simulink model "fig7_63_controleffort"  (Simulink 7.0)
settings: Solver=ode45  SolverMode=SingleTasking  StartTime=0.0  StopTime=25  RelTol=1e-3  AbsTol=1e-6
CloseFcn:
  | ;slview('closediagram',bdroot);;slview('closediagram',bdroot);
settings Model: Creator=abbas  LastModifiedBy=abbas  ExtModeTrigMode=oneshot  ExtModeArmWhenConnect=off  ExtModeAutoUpdateStatusClock=off
settings DataIOCC: LimitDataPoints=off
settings OptimizationCC: BlockReduction=off  BooleanDataType=off  InlineInvariantSignals=on
settings DebuggingCC: SaveWithParameterizedLinksMsg=none  SignalResolutionControl=TryResolveAllWithWarning  SolverPrmCheckMsg=none  MultiTaskDSMMsg=warning  MultiTaskCondExecSysMsg=none  StrictBusMsg=None
settings HardwareCC: TargetUnknown=on
settings RTWCC: IncludeERTFirstTime=on
settings GRTTargetCC: TargetFcnLib=ansi_tfl_tmw.mat  ModelReferenceCompliant=off  CompOptLevelCompliant=off  MatFileLogging=off

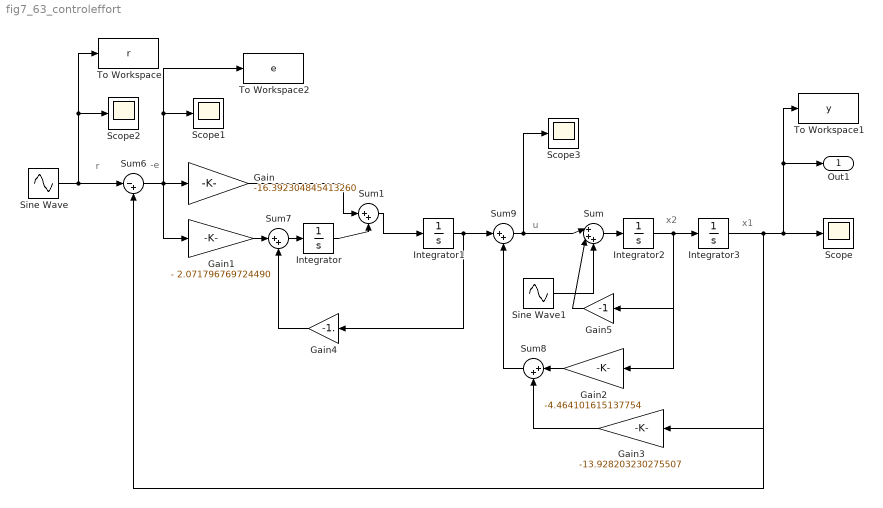
== system fig7_63_controleffort ==
  note: -e
  note: u
  note: x2
  note: x1
  note: r
  Gain : Gain  Gain=-16.392304845413260  ParameterDataType=sfix(16)  ParameterScaling=2^0  OutDataType=sfix(16)  OutScaling=2^0  SaturateOnIntegerOverflow=on
  Gain1 : Gain  Gain=- 2.071796769724490  ParameterDataType=sfix(16)  ParameterScaling=2^0  OutDataType=sfix(16)  OutScaling=2^0  SaturateOnIntegerOverflow=on
  Gain2 : Gain  Orientation=left  Gain=-4.464101615137754  ParameterDataType=sfix(16)  ParameterScaling=2^0  OutDataType=sfix(16)  OutScaling=2^0  SaturateOnIntegerOverflow=on
  Gain3 : Gain  Orientation=left  Gain=-13.928203230275507  ParameterDataType=sfix(16)  ParameterScaling=2^0  OutDataType=sfix(16)  OutScaling=2^0  SaturateOnIntegerOverflow=on
  Gain4 : Gain  Orientation=left  Gain=-1.  ParameterDataType=sfix(16)  ParameterScaling=2^0  OutDataType=sfix(16)  OutScaling=2^0  SaturateOnIntegerOverflow=on
  Gain5 : Gain  Orientation=left  Gain=-1  ParameterDataType=sfix(16)  ParameterScaling=2^0  OutDataType=sfix(16)  OutScaling=2^0  SaturateOnIntegerOverflow=on
  Integrator{,1..3} (4 alike) : Integrator
  Scope{,1..3} (4 alike) : Scope
      Scope settings: TickLabels=on  DataFormat=Array
      Scope1 settings: TickLabels=on  DataFormat=Array
      Scope3 settings: TickLabels=on  DataFormat=Array
  Sine Wave : Sin  Amplitude=0  SampleTime=.01
  Sine Wave1 : Sin  SampleTime=.01
  Sum : Sum  Inputs=|+++  OutDataType=sfix(16)  OutScaling=2^0  SaturateOnIntegerOverflow=on  InputSameDT=on
  Sum1 : Sum  Inputs=|++  OutDataType=sfix(16)  OutScaling=2^0  SaturateOnIntegerOverflow=on  InputSameDT=on
  Sum6 : Sum  Inputs=|-+  OutDataType=sfix(16)  OutScaling=2^0  SaturateOnIntegerOverflow=on  InputSameDT=on
  Sum7 : Sum  Inputs=|++  OutDataType=sfix(16)  OutScaling=2^0  SaturateOnIntegerOverflow=on  InputSameDT=on
  Sum8 : Sum  Orientation=left  Inputs=|++  OutDataType=sfix(16)  OutScaling=2^0  SaturateOnIntegerOverflow=on  InputSameDT=on
  Sum9 : Sum  Inputs=|++  OutDataType=sfix(16)  OutScaling=2^0  SaturateOnIntegerOverflow=on  InputSameDT=on
  To Workspace : ToWorkspace  VariableName=r  SampleTime=.01  SaveFormat=Array
  To Workspace1 : ToWorkspace  VariableName=y  SampleTime=0.01  SaveFormat=Array
  To Workspace2 : ToWorkspace  VariableName=e  SampleTime=0.01  SaveFormat=Array
  Out1 : Outport  OutDataType=sfix(16)  OutScaling=2^0
  wires:
  Sum7/1 -> Integrator/1
  Gain/1 -> Sum1/1
  Sum1/1 -> Integrator1/1
  Sum/1 -> Integrator2/1
  Sum6/1 -> Gain/1, Gain1/1, Scope1/1, To Workspace2/1
  Integrator3/1 -> Sum6/2, Scope/1, Out1/1, To Workspace1/1, Gain3/1
  Gain3/1 -> Sum8/2
  Gain2/1 -> Sum8/1
  Gain1/1 -> Sum7/1
  Sum8/1 -> Sum9/2
  Integrator/1 -> Sum1/2
  Gain4/1 -> Sum7/2
  Gain5/1 -> Sum/2
  Integrator1/1 -> Gain4/1, Sum9/1
  Sine Wave/1 -> Sum6/1, Scope2/1, To Workspace/1
  Sum9/1 -> Sum/1, Scope3/1
  Integrator2/1 -> Gain5/1, Gain2/1, Integrator3/1
  Sine Wave1/1 -> Sum/3
